simulink model "Traverse_mulecola"  (R2022b)
settings: Solver=VariableStepAuto  StartTime=0.0  StopTime=10.0  RelTol=1e-3
model workspace: external: MAT-File /Volumes/GoogleDrive-109291776148936580851/תיקיות אחסון שיתופי/פרויקט גמר/שלב א'/Project_main/Workspace_Project.mat (data not in the file)
undefined symbols (not defined in the file or in its folder): fix_constt, fric_gear, JLrtg, JLrtt, JMrtg, JMrtt, Kktt, Kvtt
settings Model: Creator=ohadformanair  LastModifiedBy=ohadformanair
settings DataIOCC: SaveFormat=StructureWithTime
settings OptimizationCC: BlockReduction=off  OptimizeBlockIOStorage=off  BufferReuse=off
settings ModelReferenceCC: EnableRefExpFcnMdlSchedulingChecks=on

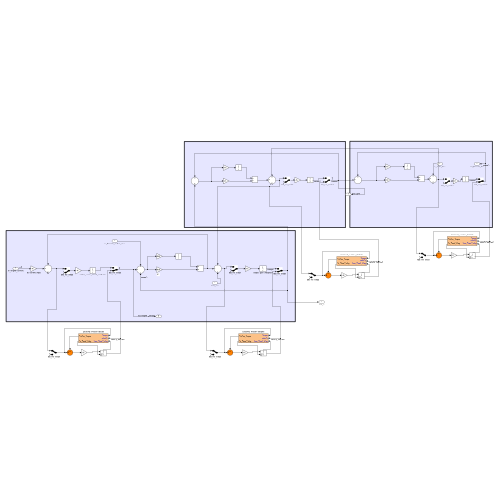
[thumbnail: Simulink's stored preview of the top-level diagram]
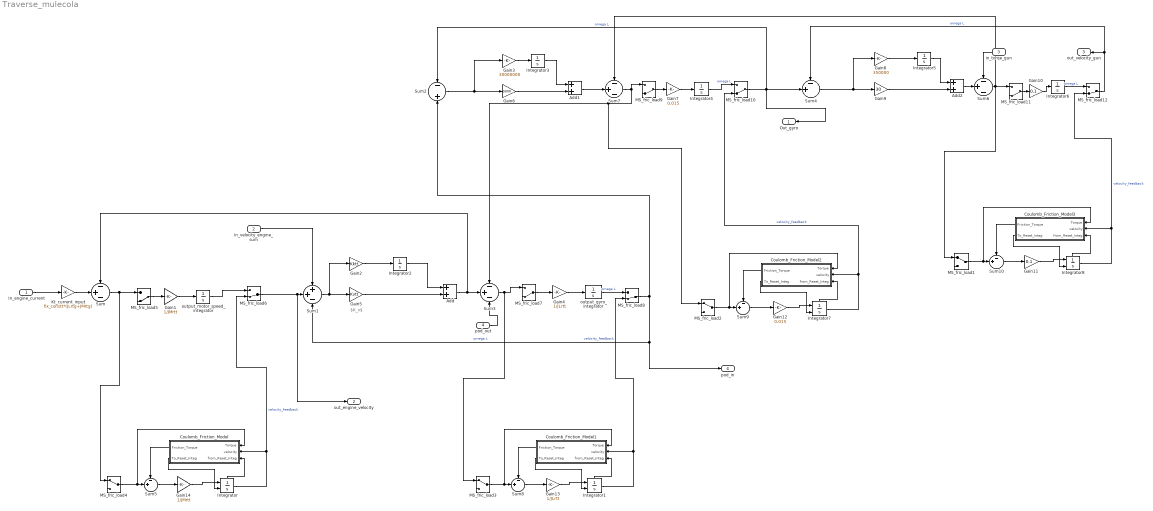
== system Traverse_mulecola ==
  note: $K_v$
  In_engine_current : Inport
  In_velocity_engine_sum : Inport  Port=2
  in_torqe_gun : Inport  Port=3
  pod_out : Inport  Port=4
  Add : Sum
  Add1 : Sum
  Add2 : Sum
  Coulomb_Friction_Model : Subsystem
  Coulomb_Friction_Model1 : Subsystem
  Coulomb_Friction_Model2 : Subsystem
  Coulomb_Friction_Model3 : Subsystem
  Gain1 : Gain  Gain=1/JMrtt
  Gain10 : Gain  Gain=0.1
  Gain11 : Gain  Gain=0.1
  Gain12 : Gain  Gain=0.015
  Gain13 : Gain  Gain=1/JLrtt
  Gain14 : Gain  Gain=1/JMrtt
  Gain2 : Gain  Gain=Kktt
  Gain3 : Gain  Gain=30000000
  Gain4 : Gain  Gain=1/JLrtt
  Gain5 : Gain  Gain=Kvtt
  Gain6 : Gain  Gain=5000
  Gain7 : Gain  Gain=0.015
  Gain8 : Gain  Gain=350000
  Gain9 : Gain  Gain=30
  Integrator{,1,7..8} (4 alike) : Integrator  ExternalReset=rising  ShowStatePort=on
  Integrator{2..6} (5 alike) : Integrator
  Kt_current_input : Gain  Gain=fix_constt*(JLrtg+JMrtg)
  MS_fric_load{1..4} (4 alike) : ManualSwitch
  MS_fric_load{5..12} (8 alike) : ManualSwitch  CurrentSetting=0
  Sum{,3,6..7} (4 alike) : Sum  Inputs=-+-
  Sum1 : Sum  Inputs=++-
  Sum{5,8..10} (4 alike) : Sum  Inputs=-+|  SaturateOnIntegerOverflow=on
  Sum2 : Sum  Inputs=-+
  Sum4 : Sum  Inputs=-+|
  output_gyro_integrator : Integrator
  output_motor_speed_integrator : Integrator
  Out_gyro : Outport
  out_engine_velocity : Outport  Port=2
  out_velocity_gun : Outport  Port=3
  pod_in : Outport  Port=4
  wires:
  In_engine_current/1 -> Kt_current_input/1
  Add1/1 -> Sum7/2
  Gain4/1 -> output_gyro_integrator/1
  Sum7/1 -> MS_fric_load9/1, MS_fric_load2/1, Sum3/1
  Gain8/1 -> Integrator5/1
  Gain7/1 -> Integrator4/1
  Sum6/1 -> MS_fric_load1/1, Sum7/1, MS_fric_load11/1
  Integrator3/1 -> Add1/1
  Gain3/1 -> Integrator3/1
  Sum3/1 -> MS_fric_load3/1, MS_fric_load7/1
  Sum1/1 -> Gain2/1, Gain5/1
  Integrator5/1 -> Add2/1
  Integrator2/1 -> Add/1
  Gain9/1 -> Add2/2
  Gain6/1 -> Add1/2
  Sum4/1 -> Gain9/1, Gain8/1
  Kt_current_input/1 -> Sum/2
  Gain2/1 -> Integrator2/1
  Gain1/1 -> output_motor_speed_integrator/1
  Add/1 -> Sum3/2, Sum/1
  Gain10/1 -> Integrator6/1
  Add2/1 -> Sum6/2
  Sum2/1 -> Gain6/1, Gain3/1
  MS_fric_load6/1 -> out_engine_velocity/1, Sum1/2
  Gain5/1 -> Add/2
  In_velocity_engine_sum/1 -> Sum1/1
  in_torqe_gun/1 -> Sum6/1
  MS_fric_load12/1 -> out_velocity_gun/1, Sum4/1  "omega L"
  MS_fric_load10/1 -> Out_gyro/1, Sum2/1, Sum4/2  "omega L"
  MS_fric_load8/1 -> Sum2/2, pod_in/1, Sum1/3  "omega L"
  Sum5/1 -> Gain14/1
  Integrator/State -> Coulomb_Friction_Model/3(from_Reset_Integ)
  Integrator/1 -> Coulomb_Friction_Model/2(velocity), MS_fric_load6/2  "velocity_feedback"
  MS_fric_load4/1 -> Coulomb_Friction_Model/1(Torque), Sum5/2
  Coulomb_Friction_Model/2(To_Reset_Integ) -> Integrator/2
  Coulomb_Friction_Model/1(Friction_Torque) -> Sum5/1
  Sum/1 -> MS_fric_load4/1, MS_fric_load5/1
  MS_fric_load5/1 -> Gain1/1
  output_motor_speed_integrator/1 -> MS_fric_load6/1
  Gain14/1 -> Integrator/1
  MS_fric_load7/1 -> Gain4/1
  output_gyro_integrator/1 -> MS_fric_load8/1  "omega L"
  Sum8/1 -> Gain13/1
  Coulomb_Friction_Model1/1(Friction_Torque) -> Sum8/1
  MS_fric_load3/1 -> Coulomb_Friction_Model1/1(Torque), Sum8/2
  Coulomb_Friction_Model1/2(To_Reset_Integ) -> Integrator1/2
  Integrator1/State -> Coulomb_Friction_Model1/3(from_Reset_Integ)
  Integrator1/1 -> MS_fric_load8/2, Coulomb_Friction_Model1/2(velocity)  "velocity_feedback"
  Gain13/1 -> Integrator1/1
  MS_fric_load9/1 -> Gain7/1
  Integrator4/1 -> MS_fric_load10/1  "omega L"
  MS_fric_load2/1 -> Coulomb_Friction_Model2/1(Torque), Sum9/2
  Sum9/1 -> Gain12/1
  Coulomb_Friction_Model2/1(Friction_Torque) -> Sum9/1
  Integrator7/1 -> MS_fric_load10/2, Coulomb_Friction_Model2/2(velocity)  "velocity_feedback"
  Integrator7/State -> Coulomb_Friction_Model2/3(from_Reset_Integ)
  Coulomb_Friction_Model2/2(To_Reset_Integ) -> Integrator7/2
  Gain12/1 -> Integrator7/1
  MS_fric_load11/1 -> Gain10/1
  Integrator6/1 -> MS_fric_load12/1  "omega L"
  Sum10/1 -> Gain11/1
  Coulomb_Friction_Model3/1(Friction_Torque) -> Sum10/1
  Gain11/1 -> Integrator8/1
  Integrator8/1 -> MS_fric_load12/2, Coulomb_Friction_Model3/2(velocity)  "velocity_feedback"
  MS_fric_load1/1 -> Coulomb_Friction_Model3/1(Torque), Sum10/2
  Integrator8/State -> Coulomb_Friction_Model3/3(from_Reset_Integ)
  Coulomb_Friction_Model3/2(To_Reset_Integ) -> Integrator8/2
  pod_out/1 -> Sum3/3

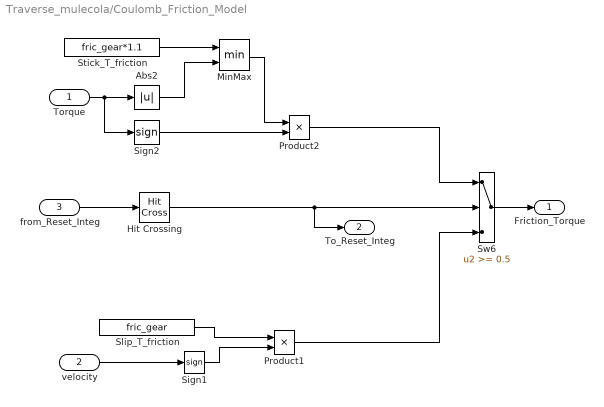
== system Traverse_mulecola/Coulomb_Friction_Model ==
  Torque : Inport
  velocity : Inport  Port=2
  from_Reset_Integ : Inport  Port=3
  Abs2 : Abs  SaturateOnIntegerOverflow=off
  Hit Crossing : HitCross  ZeroCross=off
  MinMax : MinMax  Inputs=2
  Product1 : Product  RndMeth=Zero
  Product2 : Product  RndMeth=Zero
  Sign1 : Signum  ZeroCross=off
  Sign2 : Signum  ZeroCross=off
  Slip_T_friction : Constant  Value=fric_gear
  Stick_T_friction : Constant  Value=fric_gear*1.1
  Sw6 : Switch  Threshold=0.5
  Friction_Torque : Outport
  To_Reset_Integ : Outport  Port=2
  wires:
  Torque/1 -> Abs2/1, Sign2/1
  Sw6/1 -> Friction_Torque/1
  velocity/1 -> Sign1/1
  Sign1/1 -> Product1/2
  Product1/1 -> Sw6/3
  Hit Crossing/1 -> To_Reset_Integ/1, Sw6/2
  from_Reset_Integ/1 -> Hit Crossing/1
  Sign2/1 -> Product2/2
  Stick_T_friction/1 -> MinMax/1
  Abs2/1 -> MinMax/2
  MinMax/1 -> Product2/1
  Product2/1 -> Sw6/1
  Slip_T_friction/1 -> Product1/1

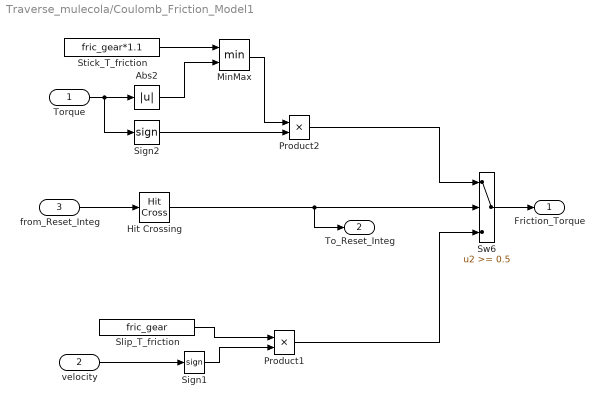
== system Traverse_mulecola/Coulomb_Friction_Model1 ==
  Torque : Inport
  velocity : Inport  Port=2
  from_Reset_Integ : Inport  Port=3
  Abs2 : Abs  SaturateOnIntegerOverflow=off
  Hit Crossing : HitCross  ZeroCross=off
  MinMax : MinMax  Inputs=2
  Product1 : Product  RndMeth=Zero
  Product2 : Product  RndMeth=Zero
  Sign1 : Signum  ZeroCross=off
  Sign2 : Signum  ZeroCross=off
  Slip_T_friction : Constant  Value=fric_gear
  Stick_T_friction : Constant  Value=fric_gear*1.1
  Sw6 : Switch  Threshold=0.5
  Friction_Torque : Outport
  To_Reset_Integ : Outport  Port=2
  wires:
  Torque/1 -> Abs2/1, Sign2/1
  Sw6/1 -> Friction_Torque/1
  velocity/1 -> Sign1/1
  Sign1/1 -> Product1/2
  Product1/1 -> Sw6/3
  Hit Crossing/1 -> To_Reset_Integ/1, Sw6/2
  from_Reset_Integ/1 -> Hit Crossing/1
  Sign2/1 -> Product2/2
  Stick_T_friction/1 -> MinMax/1
  Abs2/1 -> MinMax/2
  MinMax/1 -> Product2/1
  Product2/1 -> Sw6/1
  Slip_T_friction/1 -> Product1/1

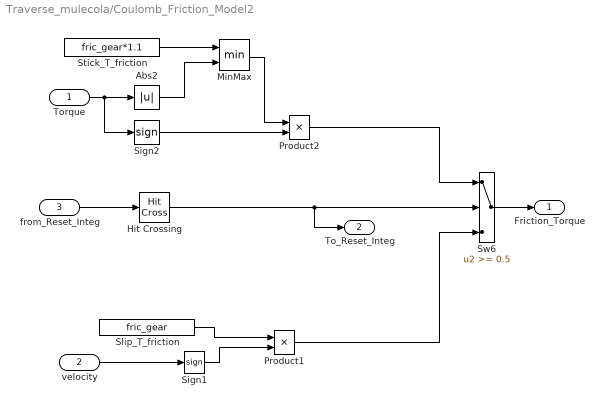
== system Traverse_mulecola/Coulomb_Friction_Model2 ==
  Torque : Inport
  velocity : Inport  Port=2
  from_Reset_Integ : Inport  Port=3
  Abs2 : Abs  SaturateOnIntegerOverflow=off
  Hit Crossing : HitCross  ZeroCross=off
  MinMax : MinMax  Inputs=2
  Product1 : Product  RndMeth=Zero
  Product2 : Product  RndMeth=Zero
  Sign1 : Signum  ZeroCross=off
  Sign2 : Signum  ZeroCross=off
  Slip_T_friction : Constant  Value=fric_gear
  Stick_T_friction : Constant  Value=fric_gear*1.1
  Sw6 : Switch  Threshold=0.5
  Friction_Torque : Outport
  To_Reset_Integ : Outport  Port=2
  wires:
  Torque/1 -> Abs2/1, Sign2/1
  Sw6/1 -> Friction_Torque/1
  velocity/1 -> Sign1/1
  Sign1/1 -> Product1/2
  Product1/1 -> Sw6/3
  Hit Crossing/1 -> To_Reset_Integ/1, Sw6/2
  from_Reset_Integ/1 -> Hit Crossing/1
  Sign2/1 -> Product2/2
  Stick_T_friction/1 -> MinMax/1
  Abs2/1 -> MinMax/2
  MinMax/1 -> Product2/1
  Product2/1 -> Sw6/1
  Slip_T_friction/1 -> Product1/1

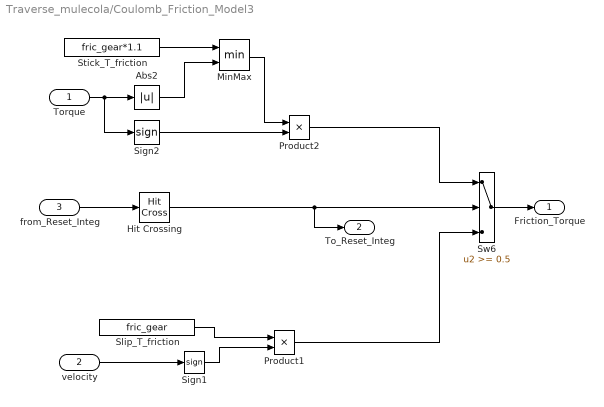
== system Traverse_mulecola/Coulomb_Friction_Model3 ==
  Torque : Inport
  velocity : Inport  Port=2
  from_Reset_Integ : Inport  Port=3
  Abs2 : Abs  SaturateOnIntegerOverflow=off
  Hit Crossing : HitCross  ZeroCross=off
  MinMax : MinMax  Inputs=2
  Product1 : Product  RndMeth=Zero
  Product2 : Product  RndMeth=Zero
  Sign1 : Signum  ZeroCross=off
  Sign2 : Signum  ZeroCross=off
  Slip_T_friction : Constant  Value=fric_gear
  Stick_T_friction : Constant  Value=fric_gear*1.1
  Sw6 : Switch  Threshold=0.5
  Friction_Torque : Outport
  To_Reset_Integ : Outport  Port=2
  wires:
  Torque/1 -> Abs2/1, Sign2/1
  Sw6/1 -> Friction_Torque/1
  velocity/1 -> Sign1/1
  Sign1/1 -> Product1/2
  Product1/1 -> Sw6/3
  Hit Crossing/1 -> To_Reset_Integ/1, Sw6/2
  from_Reset_Integ/1 -> Hit Crossing/1
  Sign2/1 -> Product2/2
  Stick_T_friction/1 -> MinMax/1
  Abs2/1 -> MinMax/2
  MinMax/1 -> Product2/1
  Product2/1 -> Sw6/1
  Slip_T_friction/1 -> Product1/1
